simulink model "SSB_TC_Receiver_1"  (R2022a)
settings: Solver=FixedStepDiscrete  StartTime=0.0  StopTime=inf  RelTol=1e-3
libraries: dspvision x2, dspsnks4 x1, dsparch4 x1, dspsigops x1, dspsrcs4 x1, matrix_library x1
settings Model: Creator=vovan  LastModifiedBy=vovan

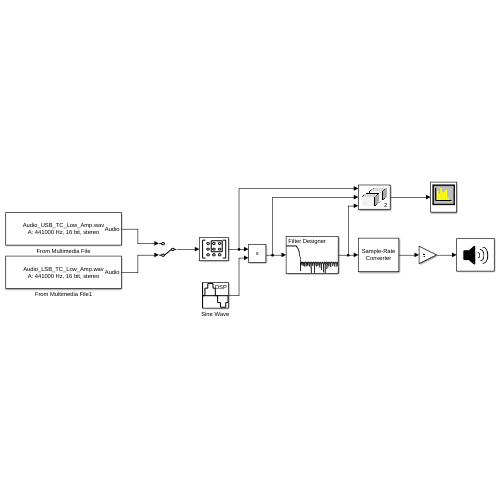
[thumbnail: Simulink's stored preview of the top-level diagram]
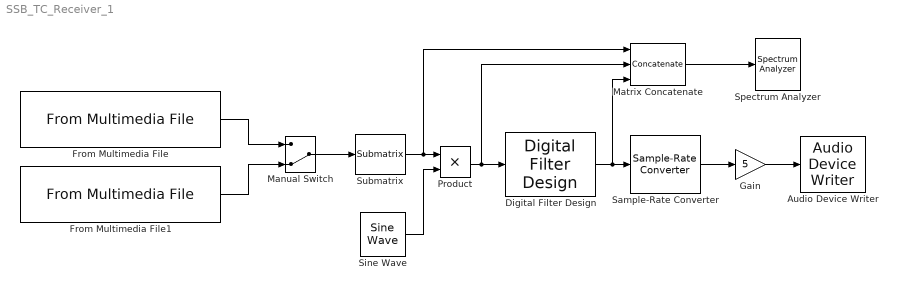
== system SSB_TC_Receiver_1 ==
  Audio Device Writer : dspsnks4/Audio Device Writer  Driver=ALSA  Device=Default  InheritSampleRate=on  SampleRate=44100  BitDepth=16-bit integer  BufferSize=4096  NumBuffers=10  DefaultOutputChannelMapping=on  OutputChannelMapping=1:2  OutputNumUnderrunSamples=off  DriverIdx=8  DeviceWarnFlag=''
  Digital Filter Design : dsparch4/Digital Filter Design  mwdsp_browser_bugfix_var=off
  From Multimedia File : dspvision/From Multimedia File  inputFilename=wav/Audio_USB_TC_Low_Amp.wav  readRange=[1 Inf]  loop=on  numPlays=inf  outputStreams=Audio only  videoDataType=single  audioDataType=double  inheritSampleTime=on  userDefinedSampleTime=1/30  noAudioOutput=off  isIntensityVideo=off  fourcc=RGB  colorVideoFormat=Separate color signals  outputEOF=off  dataOrg=Column-major  audioFrameSize=10000  computeAudioFrameSize=off  outSamplingMode=Sample based
  From Multimedia File1 : dspvision/From Multimedia File  inputFilename=wav/Audio_LSB_TC_Low_Amp.wav  readRange=[1 Inf]  loop=on  numPlays=inf  outputStreams=Audio only  videoDataType=single  audioDataType=double  inheritSampleTime=on  userDefinedSampleTime=1/30  noAudioOutput=off  isIntensityVideo=off  fourcc=RGB  colorVideoFormat=Separate color signals  outputEOF=off  dataOrg=Column-major  audioFrameSize=10000  computeAudioFrameSize=off  outSamplingMode=Sample based
  Gain : Gain  Gain=5
  Manual Switch : ManualSwitch  CurrentSetting=0
  Matrix Concatenate : Concatenate  NumInputs=3  Mode=Multidimensional array  ConcatenateDimension=2
  Product : Product
  Sample-Rate Converter : dspsigops/Sample-Rate Converter  InputSampleRate=441000  OutputSampleRate=44100  OutputRateTolerance=0  Bandwidth=40e3  StopbandAttenuation=80  SimulateUsing=Code generation
      settings: SourceProductBaseCode=DS
  Sine Wave : dspsrcs4/Sine Wave  Amplitude=1  Frequency=60e3  Phase=pi/2  SampleMode=Discrete  OutComplex=Real  CompMethod=Trigonometric fcn  TableSize=Speed  SampleTime=1/441000  SamplesPerFrame=10000  ResetState=Restart at time zero  OutputFrames=off  dataType=double  wordLen=16  udDataType=sfix(16)  fracBitsMode=Best precision  numFracBits=15  OutDataTypeStr=double  LastOutDataTypeStr=double
  Spectrum Analyzer : SpectrumAnalyzer
  Submatrix : matrix_library/Submatrix  RowSpan=All rows  RowStartMode=First  RowStartIndex=1  RowEndMode=Last  RowEndIndex=1  ColSpan=Range of columns  ColStartMode=First  ColStartIndex=1  ColEndMode=Index  ColEndIndex=1
      settings: SourceProductBaseCode=SL
  wires:
  Manual Switch/1 -> Submatrix/1
  Submatrix/1 -> Matrix Concatenate/1, Product/1
  Sine Wave/1 -> Product/2
  Product/1 -> Matrix Concatenate/2, Digital Filter Design/1
  Digital Filter Design/1 -> Matrix Concatenate/3, Sample-Rate Converter/1
  Sample-Rate Converter/1 -> Gain/1
  Gain/1 -> Audio Device Writer/1
  Matrix Concatenate/1 -> Spectrum Analyzer/1
  From Multimedia File/1 -> Manual Switch/1
  From Multimedia File1/1 -> Manual Switch/2
